simulink model "Chap7_2sim"  (R2019a)
settings: Solver=VariableStepAuto  StartTime=0.0  StopTime=30  MaxStep=.01  RelTol=1e-3
settings Model: Creator=zkibria  LastModifiedBy=zkibria

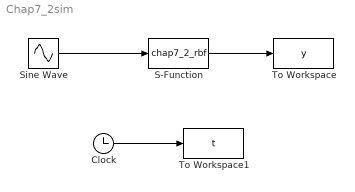
== system Chap7_2sim ==
  Clock : Clock
  S-Function : S-Function  FunctionName=chap7_2_rbf  SFunctionDeploymentMode=off  EnableBusSupport=off
  Sine Wave : Sin  SampleTime=0
  To Workspace : ToWorkspace  VariableName=y  SaveFormat=Timeseries  SampleTime=-1
  To Workspace1 : ToWorkspace  VariableName=t  SaveFormat=Timeseries  SampleTime=-1
  wires:
  S-Function/1 -> To Workspace/1
  Clock/1 -> To Workspace1/1
  Sine Wave/1 -> S-Function/1
